simulink model "r_controller_d2"  (R2024a)
settings: Solver=ode23tb  StartTime=0.0  StopTime=10.0  FixedStep=1e-5  MaxStep=1e-5  RelTol=1e-3
settings Model: Creator=PME406_01  LastModifiedBy=PME406_01

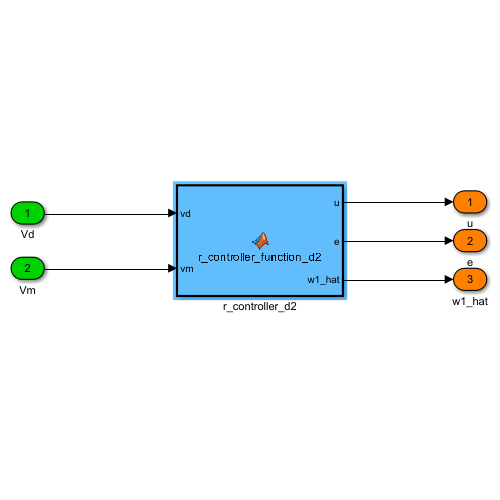
[thumbnail: Simulink's stored preview of the top-level diagram]
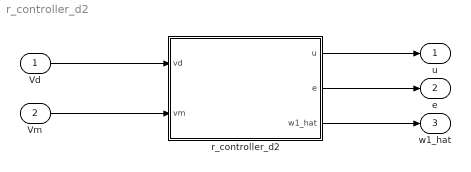
== system r_controller_d2 ==
  Vd : Inport
  Vm : Inport  Port=2
  r_controller_d2 : MATLAB Function  TreatAsAtomicUnit=on
  u : Outport
  e : Outport  Port=2
  w1_hat : Outport  Port=3
  wires:
  Vd/1 -> r_controller_d2/1(vd)
  Vm/1 -> r_controller_d2/2(vm)
  r_controller_d2/1(u) -> u/1
  r_controller_d2/2(e) -> e/1
  r_controller_d2/3(w1_hat) -> w1_hat/1

== matlab function r_controller_d2/r_controller_d2 ==
  settings: updateMethod=DISCRETE  sampleTime=1e-5
  data: vd input size=6; u output size=6; vm input size=6; e output size=6; w1_hat output size=6
function [u, e, w1_hat] = r_controller_function_d2(vd, vm)
    % R Controller with d=2 Preview (Flux_Control_R_newmodel.pdf Page 1)
    %
    % 完全平移時序方案：所有估測器公式從 k+1 平移到 k
    % 輸入：
    %   vd - 參考電壓向量 [6×1]（需要外部提供 3 步 preview）
    %   vm - 測量電壓向量 [6×1]
    % 輸出：
    %   u      - 控制輸入向量 [6×1]
    %   e      - 追蹤誤差向量 [6×1]（定義為 δv[k]）
    %   w1_hat - 干擾估測向量 [6×1]（用於監測干擾大小）
    %
    % Author: Claude Code
    % Date: 2025-10-16
    % Reference: Flux_Control_R_newmodel.pdf Page 1

    % ═══════════════════════════════════════════════════════════════════
    %                    SECTION 1: 參數定義
    % ═══════════════════════════════════════════════════════════════════

    % --- 系統模型參數 (from H(z^-1)) ---
    k_o = 5.6695e-4;              % k_o from H(z^-1)
    b = 0.9782;                   % b from H(z^-1)
    a1 = 1.934848;                % a1
    a2 = -0.935970;               % a2

    % --- B 矩陣 (6×6) ---
    B = [0.2365  -0.0064  -0.0327  -0.0344  -0.0408  -0.0343;
        -0.0037   0.2818  -0.0427  -0.0675  -0.0779  -0.0368;
        -0.0375  -0.0328   0.2108  -0.0060  -0.0265  -0.0341;
        -0.0245  -0.0777  -0.0056   0.2361  -0.0770  -0.0241;
        -0.0413  -0.0760  -0.0234  -0.0720   0.2572  -0.0045;
        -0.0244  -0.0330  -0.0257  -0.0245  -0.0030   0.1845];

    % --- B 反矩陣 ---
    B_inv = inv(B);

    % --- 控制參數 ---
    lambda_c = 0.8179;            % λc - 控制器特徵值
    lambda_e = 0.3659;            % λe - 估測器特徵值
    beta = lambda_c^2;            % β

    % --- 派生參數 ---
    kc = (1 - lambda_c) / (1 + b);
    bc = b * kc;
    ku = kc / k_o;

    % --- 估測器增益 ---
    % ℓ1
    l_1 = lambda_c + (1 + beta) - 3*lambda_e;

    % ℓ2
    l_2 = (b*(lambda_e - 1)^3 - beta*(b + 1)*(beta^2 - 3*beta*lambda_e + beta + 3*lambda_e^2 - 3*lambda_e + 1)) / ...
          (kc * (b + 1) * (b + beta));

    % ℓ3
    l_3 = (-(b + beta)*(beta^2 - 3*beta*lambda_e + beta + 3*lambda_e^2 - 3*lambda_e + 1) - lambda_e^3) / ...
          (kc * (b + 1) * (b + beta));

    % ═══════════════════════════════════════════════════════════════════
    %              SECTION 2: Persistent 變數聲明與初始化
    % ═══════════════════════════════════════════════════════════════════

    % --- VD Buffer (d=2 需要 4 層) ---
    persistent vd_buffer          % vd buffer: [vd[k]; vd[k+1]; vd[k+2]; vd[k+3]]

    % --- VF 預濾波器歷史 ---
    persistent vf                 % vf[k] - 當前時刻
    persistent vf_k1              % vf[k-1] - 過去 1 步

    % --- 增量歷史 ---
    persistent delta_vf_k1        % δvf[k-1]
    persistent delta_v_k1         % δv[k-1]

    % --- 估測器狀態歷史 ---
    persistent delta_v_hat_k1     % δv̂[k-1]
    persistent w1_hat_k1          % ŵ1[k-1]
    persistent w2_hat_k1          % ŵ2[k-1]

    % --- 控制律歷史 ---
    persistent uc_k1              % uc[k-1]
    persistent uc_k2              % uc[k-2]
    persistent delta_vc_k1        % δvc[k-1]
    persistent delta_vc_k2        % δvc[k-2]

    % --- 初始化標誌 ---
    persistent initialized

    if isempty(initialized)
        initialized = true;

        % Buffer 初始化（4 層：k, k+1, k+2, k+3）
        vd_buffer = zeros(4, 6);  % Row 1: vd[k], Row 2: vd[k+1], Row 3: vd[k+2], Row 4: vd[k+3]

        % VF 濾波器初始化
        vf = zeros(6, 1);
        vf_k1 = zeros(6, 1);

        % 增量初始化
        delta_vf_k1 = zeros(6, 1);
        delta_v_k1 = zeros(6, 1);

        % 估測器初始化
        delta_v_hat_k1 = zeros(6, 1);
        w1_hat_k1 = zeros(6, 1);
        w2_hat_k1 = zeros(6, 1);

        % 控制律初始化
        uc_k1 = zeros(6, 1);
        uc_k2 = zeros(6, 1);
        delta_vc_k1 = zeros(6, 1);
        delta_vc_k2 = zeros(6, 1);
    end

    % ═══════════════════════════════════════════════════════════════════
    %                SECTION 3: VD Buffer 管理 (d=2)
    % ═══════════════════════════════════════════════════════════════════

    % Buffer 更新：vd[k] <- vd[k+1] <- vd[k+2] <- vd[k+3] <- new input
    vd_buffer(1, :) = vd_buffer(2, :);  % vd[k] = old vd[k+1]
    vd_buffer(2, :) = vd_buffer(3, :);  % vd[k+1] = old vd[k+2]
    vd_buffer(3, :) = vd_buffer(4, :);  % vd[k+2] = old vd[k+3]
    vd_buffer(4, :) = vd';              % vd[k+3] = new input (假設外部已 preview)

    % 提取各時刻的 vd（轉置為列向量）
    vd_k        = vd_buffer(1, :)';  % vd[k] - 當前時刻
    vd_k_plus1  = vd_buffer(2, :)';  % vd[k+1] - preview 1 步
    vd_k_plus2  = vd_buffer(3, :)';  % vd[k+2] - preview 2 步
    vd_k_plus3  = vd_buffer(4, :)';  % vd[k+3] - preview 3 步

    % ═══════════════════════════════════════════════════════════════════
    %             SECTION 4: VF 預濾波器計算 (PDF Step 1, d=2)
    % ═══════════════════════════════════════════════════════════════════

    % vf[k+1] = 1/((1-λc)(1+b)) {b·vd[k+3] + (1-b·λc)·vd[k+2] - λc·vd[k+1]}
    vf_next = (1 / ((1 - lambda_c) * (1 + b))) * ...
              (b * vd_k_plus3 + (1 - b*lambda_c) * vd_k_plus2 - lambda_c * vd_k_plus1);

    % ═══════════════════════════════════════════════════════════════════
    %              SECTION 5: 增量計算 (PDF Step 2)
    % ═══════════════════════════════════════════════════════════════════

    % δvf[k] = vf[k+1] - (1-bc)·vf[k] - bc·vf[k-1]
    delta_vf = vf_next - (1 - bc)*vf - bc*vf_k1;

    % δv[k] = vf[k] - vm[k]
    delta_v = vf - vm;

    % ═══════════════════════════════════════════════════════════════════
    %          SECTION 6: 估測器狀態更新 (PDF Step 3, 完全平移)
    % ═══════════════════════════════════════════════════════════════════

    % 誤差項（使用 k-1 時刻的資訊）
    error_term = delta_v_k1 - delta_v_hat_k1;

    % δv̂[k] = λc·δv̂[k-1] + δvf[k-1] + ℓ1{δv[k-1] - δv̂[k-1]}
    delta_v_hat = lambda_c * delta_v_hat_k1 + delta_vf_k1 + l_1 * error_term;

    % ŵ1[k] = (1+β)·ŵ1[k-1] - β·ŵ2[k-1] + ℓ2{δv[k-1] - δv̂[k-1]}
    w1_hat = (1 + beta) * w1_hat_k1 - beta * w2_hat_k1 + l_2 * error_term;

    % ŵ2[k] = ŵ1[k-1] + ℓ3{δv[k-1] - δv̂[k-1]}
    w2_hat = w1_hat_k1 + l_3 * error_term;

    % ═══════════════════════════════════════════════════════════════════
    %                  SECTION 7: 控制律計算 (PDF Step 4)
    % ═══════════════════════════════════════════════════════════════════

    % δvc[k] = δv[k] - ŵ1[k]
    delta_vc = delta_v - w1_hat;

    % uc[k] = (1-bc)·uc[k-1] - bc·uc[k-2] + ku·{δvc[k] - a1·δvc[k-1] - a2·δvc[k-2]}
    uc = (1 - bc) * uc_k1 - bc * uc_k2 + ...
         ku * (delta_vc - a1 * delta_vc_k1 - a2 * delta_vc_k2);

    % u[k] = B^(-1)·uc[k]
    u = B_inv * uc;

    % 輸出誤差（定義為 δv[k]）
    e = delta_v;

    % ═══════════════════════════════════════════════════════════════════
    %               SECTION 8: 歷史變數更新（為下一時刻準備）
    % ═══════════════════════════════════════════════════════════════════

    % VF 濾波器歷史更新
    vf_k1 = vf;        % vf[k-1] ← vf[k]
    vf = vf_next;      % vf[k] ← vf[k+1]

    % 增量歷史更新
    delta_vf_k1 = delta_vf;  % δvf[k-1] ← δvf[k]
    delta_v_k1 = delta_v;    % δv[k-1] ← δv[k]

    % 估測器歷史更新
    delta_v_hat_k1 = delta_v_hat;  % δv̂[k-1] ← δv̂[k]
    w1_hat_k1 = w1_hat;            % ŵ1[k-1] ← ŵ1[k]
    w2_hat_k1 = w2_hat;            % ŵ2[k-1] ← ŵ2[k]

    % 控制律歷史更新
    uc_k2 = uc_k1;              % uc[k-2] ← uc[k-1]
    uc_k1 = uc;                 % uc[k-1] ← uc[k]
    delta_vc_k2 = delta_vc_k1;  % δvc[k-2] ← δvc[k-1]
    delta_vc_k1 = delta_vc;     % δvc[k-1] ← δvc[k]
end
